simulink model "MoveMoveNewModel"  (R2018a)
settings: Solver=VariableStepAuto  StartTime=0.0  StopTime=10  RelTol=1e-3
PostLoadFcn:
  | helperSetUp
values from neighbouring files (symbols this model uses):
  bf = 12    [data_vehicle.m]    (also in matlab.mat; myVehicle.m)
  br = 14    [data_vehicle.m]    (also in matlab.mat; myVehicle.m)
  Cd = .3    (= 0.3)    [data_vehicle.m]    (also in matlab.mat; myVehicle.m = this.CD)
  Cf = 1.3    [data_vehicle.m]    (also in forwardPropagate.m = 19000; matlab.mat; myVehicle.m; testMotionPlanner.mat = 19000)
  Cr = 1.3    [data_vehicle.m]    (also in forwardPropagate.m = 33000; matlab.mat; myVehicle.m; testMotionPlanner.mat = 33000)
  df = 0.95    [data_vehicle.m]    (also in matlab.mat; myVehicle.m)
  dr = 1    [data_vehicle.m]    (also in matlab.mat; myVehicle.m)
  Ef = -0.1    [data_vehicle.m]    (also in matlab.mat; myVehicle.m)
  Er = -0.1    [data_vehicle.m]    (also in matlab.mat; myVehicle.m)
  fv = .02    (= 0.02)    [data_vehicle.m]    (also in matlab.mat; myVehicle.m)
  Fzf = m*g*lr/l    (= 9879.29185185)    [data_vehicle.m]    (also in matlab.mat; myVehicle.m = m*g*lr/l)
  Fzr = m*g*lf/l    (= 5811.34814815)    [data_vehicle.m]    (also in matlab.mat; myVehicle.m = m*g*lf/l)
  g = 9.80665    [data_vehicle.m]    (also in matlab.mat)
  gB = 2/3    (= 0.666666666667)    [data_vehicle.m]    (also in matlab.mat; myVehicle.m)
  gT = 0    [data_vehicle.m]    (also in matlab.mat; myVehicle.m)
  Jz = 2200    [data_vehicle.m]    (also in matlab.mat; myVehicle.m)
  lf = 1    [data_vehicle.m]    (also in forwardPropagate.m = 1.2; matlab.mat; myVehicle.m; testMotionPlanner.mat = 1.2)
  lr = l-lf    (= 1.7)    [data_vehicle.m]    (also in forwardPropagate.m = 1.6; matlab.mat; myVehicle.m; testMotionPlanner.mat = 1.6)
  m = 1600    [data_vehicle.m]    (also in forwardPropagate.m = 1575; matlab.mat; myVehicle.m; testMotionPlanner.mat = 1575)
  mu = 1    [data_vehicle.m]    (also in matlab.mat; myVehicle.m)
  psi0 = 0    [data_vehicle.m]    (also in matlab.mat)
  psip0 = 0    [data_vehicle.m]    (also in matlab.mat)
  rho = 1.2    [data_vehicle.m]    (also in matlab.mat; myVehicle.m = 1.29)
  S = 2    [data_vehicle.m]    (also in matlab.mat; myVehicle.m)
  vy0 = 0    [data_vehicle.m]    (also in matlab.mat)
  XG0 = 0    [data_vehicle.m]    (also in matlab.mat)
  YG0 = 0    [data_vehicle.m]    (also in matlab.mat)
undefined symbols (not defined in the file or in its folder): deltah, dt_save, fxh
settings Model: Creator=jdrjk  LastModifiedBy=jdrjk

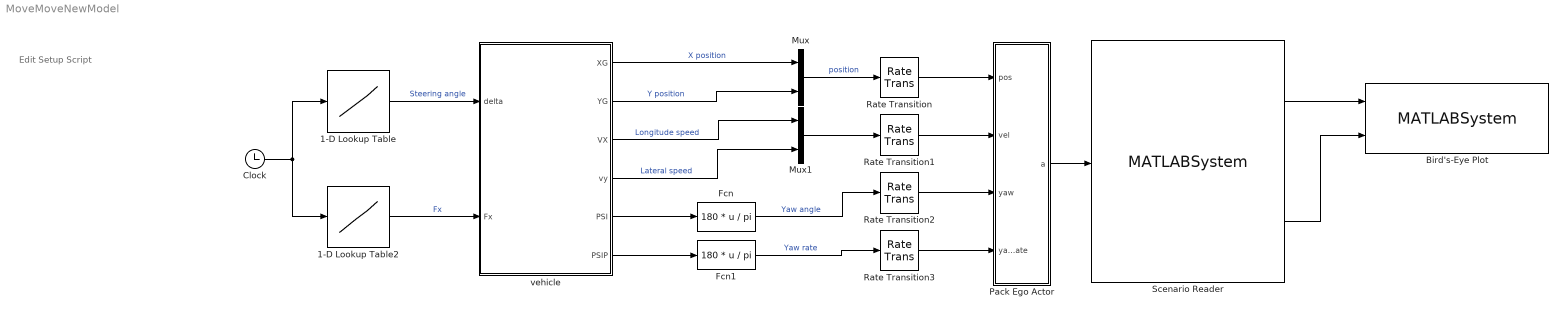
== system MoveMoveNewModel ==
  note: Edit Setup Script
  1-D Lookup Table : Lookup_n-D  NumberOfTableDimensions=1  BreakpointsForDimension1=deltah(:,1)  Table=deltah(:,2)  RndMeth=Simplest  InputSameDT=on
  1-D Lookup Table2 : Lookup_n-D  NumberOfTableDimensions=1  BreakpointsForDimension1=fxh(:,1)  Table=fxh(:,2)  RndMeth=Simplest  InputSameDT=on
  Bird's-Eye Plot : MATLABSystem  System=helperBirdsEyePlot  ScenarioFileName=lkaScenarioSimulink  XLim=[-20, 50 ]  YLim=[ -30, 30 ]  HasActors=on  HasVision=off  HasRadar=off  HasTracks=off  TrackPositionSelector=[ 1, 0, 0, 0, 0, 0; 0, 0, 1, 0, 0, 0 ]  TrackVelocitySelector=[ 0, 1, 0, 0, 0, 0; 0, 0, 0, 1, 0, 0 ]  HasMIO=off  HasRoads=off  HasLaneBoundaries=off  HasLaneMarkings=on
      settings: ModelCloseFcn=helperCloseAll(gcb)
      mask Type: helperBirdsEyePlot
      mask Display:
      | disp(['Bird''s-Eye' char(10) 'Plot']);
      | port_label('input',1,'Actors');
      | port_label('input',2,'Lane Markings');
  Clock : Clock
  Fcn : Fcn  Expr=180 * u / pi
  Fcn1 : Fcn  Expr=180 * u / pi
  Mux : Mux  Inputs=2
  Mux1 : Mux  Inputs=2
  Pack Ego Actor : MATLAB Function  TreatAsAtomicUnit=on
  Rate Transition{,1..3} (4 alike) : RateTransition  OutPortSampleTime=Ts
  Scenario Reader : MATLABSystem  System=helperScenarioReader  ScenarioFileName=lkaScenarioSimulink  EgoActorSource=Input port  EgoActorID=1  RoadBoundaries=off  LaneBoundaries=off  AllBoundaries=off  LaneBoundaryDistance=0:0.5:60  LaneBoundaryLocation=inner  CurrentLane=off  NumLanes=off  LaneMarkings=on  BusNameSource=Auto  BusName2Source=Auto  BusName3Source=Auto  SimulateUsing=Interpreted execution
      mask Type: helperScenarioReader
      mask Display:
      | disp(['Scenario' char(10) 'Reader']);
      | port_label('input',1,'Ego Actor');
      | port_label('output',1,'Actors');
      | port_label('output',2,'Lane Markings');
  vehicle : Subsystem
  wires:
  Rate Transition2/1 -> Pack Ego Actor/3(yaw)
  Mux1/1 -> Rate Transition1/1
  Rate Transition/1 -> Pack Ego Actor/1(pos)
  Scenario Reader/1 -> Bird's-Eye Plot/1
  Fcn1/1 -> Rate Transition3/1  "Yaw rate"
  Mux/1 -> Rate Transition/1  "position"
  Pack Ego Actor/1(a) -> Scenario Reader/1
  Rate Transition3/1 -> Pack Ego Actor/4(yawRate)
  Rate Transition1/1 -> Pack Ego Actor/2(vel)
  Fcn/1 -> Rate Transition2/1  "Yaw angle"
  Scenario Reader/2 -> Bird's-Eye Plot/2
  vehicle/6("PSIP ") -> Fcn1/1
  1-D Lookup Table/1 -> vehicle/1(delta)  "Steering angle"
  Clock/1 -> 1-D Lookup Table/1, 1-D Lookup Table2/1
  vehicle/5(PSI) -> Fcn/1
  vehicle/2(YG) -> Mux/2  "Y position"
  vehicle/1(XG) -> Mux/1  "X position"
  vehicle/3(VX) -> Mux1/1  "Longitude speed"
  vehicle/4(vy) -> Mux1/2  "Lateral speed"
  1-D Lookup Table2/1 -> vehicle/2("Fx ")  "Fx"

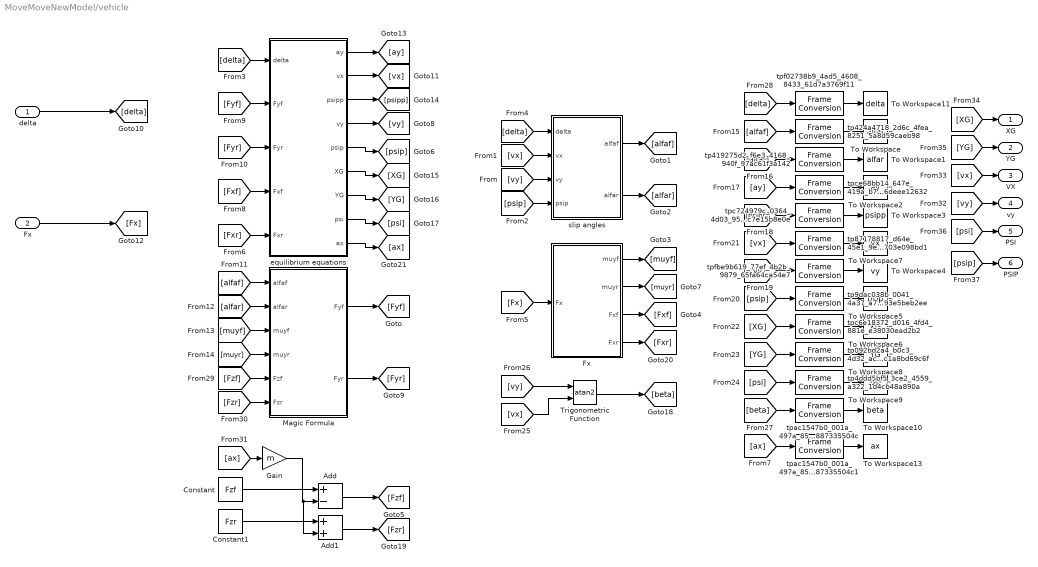
== system MoveMoveNewModel/vehicle ==
  delta : Inport
  "Fx " : Inport  Port=2
  Add : Sum  Inputs=+-
  Add1 : Sum
  Constant : Constant  Value=Fzf
  Constant1 : Constant  Value=Fzr
  Fx : Subsystem
  Gain : Gain  Gain=m
  Magic Formula : Subsystem
  To Workspace : ToWorkspace  VariableName=alfaf  SampleTime=dt_save
  To Workspace1 : ToWorkspace  VariableName=alfar  SampleTime=dt_save
  To Workspace10 : ToWorkspace  VariableName=beta  SampleTime=dt_save
  To Workspace11 : ToWorkspace  VariableName=delta  SampleTime=dt_save
  To Workspace13 : ToWorkspace  VariableName=ax  SampleTime=dt_save
  To Workspace2 : ToWorkspace  VariableName=ay  SampleTime=dt_save
  To Workspace3 : ToWorkspace  VariableName=psipp  SampleTime=dt_save
  To Workspace4 : ToWorkspace  VariableName=vy  SampleTime=dt_save
  To Workspace5 : ToWorkspace  VariableName=psip  SampleTime=dt_save
  To Workspace6 : ToWorkspace  VariableName=XG  SampleTime=dt_save
  To Workspace7 : ToWorkspace  VariableName=vx  SampleTime=dt_save
  To Workspace8 : ToWorkspace  VariableName=YG  SampleTime=dt_save
  To Workspace9 : ToWorkspace  VariableName=psi  SampleTime=dt_save
  Trigonometric Function : Trigonometry  Operator=atan2
  equilibrium equations : Subsystem
  slip angles : Subsystem
  tp092bd2a4_b0c3_4d32_ac59_7c1a8bd69c6f : FrameConversion  OutFrame=Sample-based
  tp419275d2_f6e3_4168_940f_97ac61f3a142 : FrameConversion  OutFrame=Sample-based
  tp424a4718_2d6c_4fea_8251_5a8d59caeb98 : FrameConversion  OutFrame=Sample-based
  tp4ddd5bf5_3ce2_4559_a322_1d4cb48a890a : FrameConversion  OutFrame=Sample-based
  tp87178817_d64e_45e1_9e30_db703e098bd1 : FrameConversion  OutFrame=Sample-based
  tp9dac038b_0041_4a37_a752_0593e5beb2ee : FrameConversion  OutFrame=Sample-based
  tpac1547b0_001a_497a_857c_68887335504c : FrameConversion  OutFrame=Sample-based
  tpac1547b0_001a_497a_857c_68887335504c1 : FrameConversion  OutFrame=Sample-based
  tpc6e18372_d016_4fd4_881e_e38030ead2b2 : FrameConversion  OutFrame=Sample-based
  tpc724979c_0364_4d03_952a_37c7e15b8e0e : FrameConversion  OutFrame=Sample-based
  tpce68bb14_647e_419a_b744_5f6deee12632 : FrameConversion  OutFrame=Sample-based
  tpf02738b9_4ad5_4608_8433_61d7a3769f11 : FrameConversion  OutFrame=Sample-based
  tpfbe9b619_77ef_4b2b_9879_65fa64ca54e7 : FrameConversion  OutFrame=Sample-based
  XG : Outport
  YG : Outport  Port=2
  VX : Outport  Port=3
  vy : Outport  Port=4
  PSI : Outport  Port=5
  "PSIP " : Outport  Port=6
  wires:
  [vx] -> VX/1
  [psi] -> PSI/1
  [XG] -> XG/1
  [YG] -> YG/1
  [vy] -> vy/1
  Magic Formula/2(Fyr) -> [Fyr]
  slip angles/1(alfaf) -> [alfaf]
  equilibrium equations/5(psip) -> [psip]
  [delta] -> equilibrium equations/1(delta)
  [vx] -> slip angles/2(vx)
  Fx/4(Fxr) -> [Fxr]
  [Fxf] -> equilibrium equations/4(Fxf)
  [alfar] -> Magic Formula/2(alfar)
  [muyf] -> Magic Formula/3(muyf)
  [vy] -> slip angles/3(vy)
  [muyr] -> Magic Formula/4(muyr)
  slip angles/2(alfar) -> [alfar]
  Magic Formula/1(Fyf) -> [Fyf]
  [Fyf] -> equilibrium equations/2(Fyf)
  equilibrium equations/4(vy) -> [vy]
  [psip] -> slip angles/4(psip)
  [Fyr] -> equilibrium equations/3(Fyr)
  delta/1 -> [delta]
  Fx/1(muyf) -> [muyf]
  [alfaf] -> Magic Formula/1(alfaf)
  [delta] -> slip angles/1(delta)
  Fx/2(muyr) -> [muyr]
  Fx/3(Fxf) -> [Fxf]
  [delta] -> tpf02738b9_4ad5_4608_8433_61d7a3769f11/1
  tpf02738b9_4ad5_4608_8433_61d7a3769f11/1 -> To Workspace11/1
  [ay] -> tpce68bb14_647e_419a_b744_5f6deee12632/1
  equilibrium equations/8(psi) -> [psi]
  [alfar] -> tp419275d2_f6e3_4168_940f_97ac61f3a142/1
  [alfaf] -> tp424a4718_2d6c_4fea_8251_5a8d59caeb98/1
  tpce68bb14_647e_419a_b744_5f6deee12632/1 -> To Workspace2/1
  [psipp] -> tpc724979c_0364_4d03_952a_37c7e15b8e0e/1
  equilibrium equations/3(psipp) -> [psipp]
  [vy] -> Trigonometric Function/1
  [Fzf] -> Magic Formula/5(Fzf)
  Gain/1 -> Add1/2, Add/2
  tp424a4718_2d6c_4fea_8251_5a8d59caeb98/1 -> To Workspace/1
  [beta] -> tpac1547b0_001a_497a_857c_68887335504c/1
  equilibrium equations/7(YG) -> [YG]
  Add1/1 -> [Fzr]
  tpac1547b0_001a_497a_857c_68887335504c/1 -> To Workspace10/1
  equilibrium equations/1(ay) -> [ay]
  Constant/1 -> Add/1
  equilibrium equations/6(XG) -> [XG]
  Constant1/1 -> Add1/1
  [Fzr] -> Magic Formula/6(Fzr)
  Trigonometric Function/1 -> [beta]
  Add/1 -> [Fzf]
  [vx] -> Trigonometric Function/2
  [ax] -> Gain/1
  tp419275d2_f6e3_4168_940f_97ac61f3a142/1 -> To Workspace1/1
  tp092bd2a4_b0c3_4d32_ac59_7c1a8bd69c6f/1 -> To Workspace8/1
  tp4ddd5bf5_3ce2_4559_a322_1d4cb48a890a/1 -> To Workspace9/1
  tpc724979c_0364_4d03_952a_37c7e15b8e0e/1 -> To Workspace3/1
  [psip] -> tp9dac038b_0041_4a37_a752_0593e5beb2ee/1
  tp87178817_d64e_45e1_9e30_db703e098bd1/1 -> To Workspace7/1
  tpc6e18372_d016_4fd4_881e_e38030ead2b2/1 -> To Workspace6/1
  [vy] -> tpfbe9b619_77ef_4b2b_9879_65fa64ca54e7/1
  tpfbe9b619_77ef_4b2b_9879_65fa64ca54e7/1 -> To Workspace4/1
  [XG] -> tpc6e18372_d016_4fd4_881e_e38030ead2b2/1
  [YG] -> tp092bd2a4_b0c3_4d32_ac59_7c1a8bd69c6f/1
  [vx] -> tp87178817_d64e_45e1_9e30_db703e098bd1/1
  tp9dac038b_0041_4a37_a752_0593e5beb2ee/1 -> To Workspace5/1
  [psi] -> tp4ddd5bf5_3ce2_4559_a322_1d4cb48a890a/1
  [psip] -> "PSIP "/1
  "Fx "/1 -> [Fx]
  [Fx] -> Fx/1(Fx)
  [Fxr] -> equilibrium equations/5("Fxr ")
  equilibrium equations/9(ax) -> [ax]
  [ax] -> tpac1547b0_001a_497a_857c_68887335504c1/1
  tpac1547b0_001a_497a_857c_68887335504c1/1 -> To Workspace13/1
  equilibrium equations/2("vx ") -> [vx]

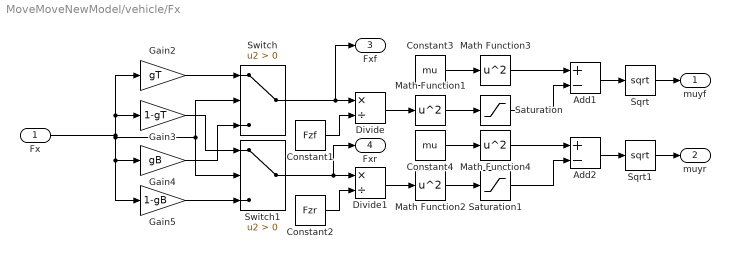
== system MoveMoveNewModel/vehicle/Fx ==
  Fx : Inport
  Add1 : Sum  Inputs=+-
  Add2 : Sum  Inputs=+-
  Constant1 : Constant  Value=Fzf
  Constant2 : Constant  Value=Fzr
  Constant3 : Constant  Value=mu
  Constant4 : Constant  Value=mu
  Divide : Product  Inputs=*/
  Divide1 : Product  Inputs=*/
  Gain2 : Gain  Gain=gT
  Gain3 : Gain  Gain=1-gT
  Gain4 : Gain  Gain=gB
  Gain5 : Gain  Gain=1-gB
  Math Function{1..4} (4 alike) : Math  Operator=square  SaturateOnIntegerOverflow=on
  Saturation : Saturate  UpperLimit=1  LowerLimit=0
  Saturation1 : Saturate  UpperLimit=1  LowerLimit=0
  Sqrt : Sqrt  SaturateOnIntegerOverflow=on
  Sqrt1 : Sqrt  SaturateOnIntegerOverflow=on
  Switch : Switch  Criteria=u2 > Threshold
  Switch1 : Switch  Criteria=u2 > Threshold
  muyf : Outport
  muyr : Outport  Port=2
  Fxf : Outport  Port=3
  Fxr : Outport  Port=4
  wires:
  Gain4/1 -> Switch/3
  Fx/1 -> Gain2/1, Gain3/1, Gain5/1, Gain4/1, Switch1/2, Switch/2
  Gain3/1 -> Switch1/1
  Gain5/1 -> Switch1/3
  Gain2/1 -> Switch/1
  Switch/1 -> Fxf/1, Divide/1
  Switch1/1 -> Fxr/1, Divide1/1
  Constant1/1 -> Divide/2
  Constant2/1 -> Divide1/2
  Constant3/1 -> Math Function3/1
  Divide/1 -> Math Function1/1
  Divide1/1 -> Math Function2/1
  Math Function1/1 -> Saturation/1
  Math Function2/1 -> Saturation1/1
  Constant4/1 -> Math Function4/1
  Saturation1/1 -> Add2/2
  Saturation/1 -> Add1/2
  Add1/1 -> Sqrt/1
  Add2/1 -> Sqrt1/1
  Sqrt1/1 -> muyr/1
  Sqrt/1 -> muyf/1
  Math Function3/1 -> Add1/1
  Math Function4/1 -> Add2/1

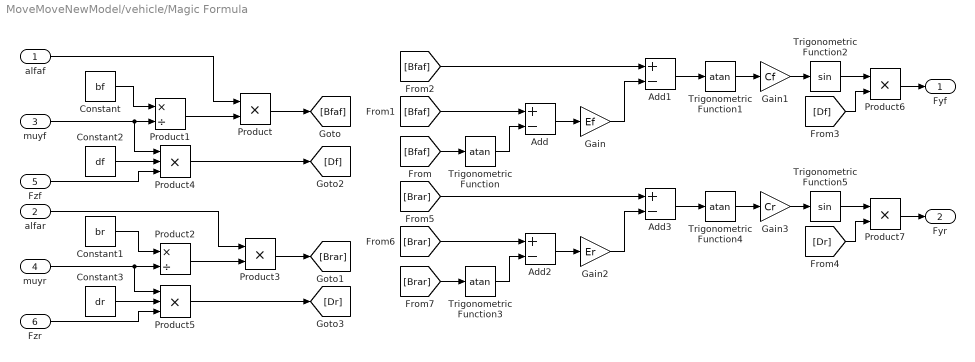
== system MoveMoveNewModel/vehicle/Magic Formula ==
  alfaf : Inport
  alfar : Inport  Port=2
  muyf : Inport  Port=3
  muyr : Inport  Port=4
  Fzf : Inport  Port=5
  Fzr : Inport  Port=6
  Add{,1..3} (4 alike) : Sum  Inputs=+-
  Constant : Constant  Value=bf
  Constant1 : Constant  Value=br
  Constant2 : Constant  Value=df
  Constant3 : Constant  Value=dr
  Gain : Gain  Gain=Ef
  Gain1 : Gain  Gain=Cf
  Gain2 : Gain  Gain=Er
  Gain3 : Gain  Gain=Cr
  Product{,3,6..7} (4 alike) : Product
  Product1 : Product  Inputs=*/
  Product2 : Product  Inputs=*/
  Product4 : Product  Inputs=3
  Product5 : Product  Inputs=3
  Trigonometric Function{,1,3..4} (4 alike) : Trigonometry  Operator=atan
  Trigonometric Function2 : Trigonometry
  Trigonometric Function5 : Trigonometry
  Fyf : Outport
  Fyr : Outport  Port=2
  wires:
  Constant/1 -> Product1/1
  muyf/1 -> Product4/1, Product1/2
  Constant1/1 -> Product2/1
  muyr/1 -> Product5/1, Product2/2
  Product1/1 -> Product/2
  alfaf/1 -> Product/1
  Product2/1 -> Product3/2
  alfar/1 -> Product3/1
  Product/1 -> [Bfaf]
  Product3/1 -> [Brar]
  Constant2/1 -> Product4/2
  Constant3/1 -> Product5/2
  Product4/1 -> [Df]
  Product5/1 -> [Dr]
  [Bfaf] -> Trigonometric Function/1
  Trigonometric Function/1 -> Add/2
  [Bfaf] -> Add/1
  Add/1 -> Gain/1
  Gain/1 -> Add1/2
  [Bfaf] -> Add1/1
  Add1/1 -> Trigonometric Function1/1
  Trigonometric Function1/1 -> Gain1/1
  Gain1/1 -> Trigonometric Function2/1
  Trigonometric Function2/1 -> Product6/1
  [Df] -> Product6/2
  Product6/1 -> Fyf/1
  [Dr] -> Product7/2
  Trigonometric Function5/1 -> Product7/1
  Gain3/1 -> Trigonometric Function5/1
  Trigonometric Function4/1 -> Gain3/1
  Add3/1 -> Trigonometric Function4/1
  [Brar] -> Add3/1
  Gain2/1 -> Add3/2
  Add2/1 -> Gain2/1
  [Brar] -> Add2/1
  Trigonometric Function3/1 -> Add2/2
  [Brar] -> Trigonometric Function3/1
  Product7/1 -> Fyr/1
  Fzf/1 -> Product4/3
  Fzr/1 -> Product5/3

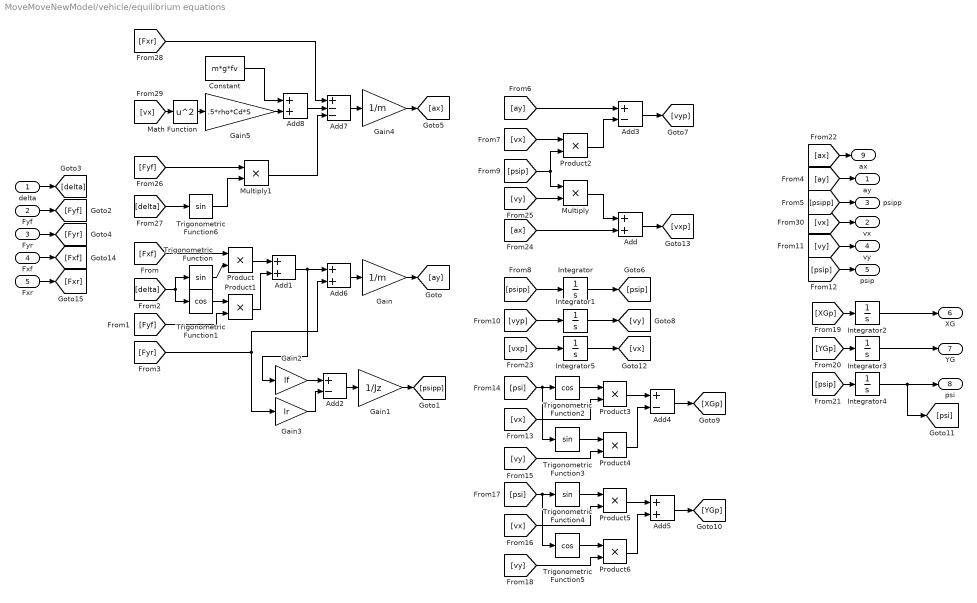
== system MoveMoveNewModel/vehicle/equilibrium equations ==
  delta : Inport
  Fyf : Inport  Port=2
  Fyr : Inport  Port=3
  Fxf : Inport  Port=4
  "Fxr " : Inport  Port=5
  Add{,1,5..6,8} (5 alike) : Sum
  Add2 : Sum  Inputs=+-
  Add3 : Sum  Inputs=+-
  Add4 : Sum  Inputs=+-
  Add7 : Sum  Inputs=+--
  Constant : Constant  Value=m*g*fv
  Gain : Gain  Gain=1/m
  Gain1 : Gain  Gain=1/Jz
  Gain2 : Gain  Gain=lf
  Gain3 : Gain  Gain=lr
  Gain4 : Gain  Gain=1/m
  Gain5 : Gain  Gain=.5*rho*Cd*S
  Integrator : Integrator  InitialCondition=psip0  ContinuousStateAttributes='yaw_rate'
  Integrator1 : Integrator  InitialCondition=vy0  ContinuousStateAttributes='speed_y'
  Integrator2 : Integrator  InitialCondition=XG0  ContinuousStateAttributes='XG'
  Integrator3 : Integrator  InitialCondition=YG0  ContinuousStateAttributes='YG'
  Integrator4 : Integrator  InitialCondition=psi0  ContinuousStateAttributes='yaw'
  Integrator5 : Integrator  InitialCondition=vy0  ContinuousStateAttributes='speed_y'
  Math Function : Math  Operator=square  SaturateOnIntegerOverflow=on
  Multiply : Product
  Multiply1 : Product
  Product{,1..6} (7 alike) : Product
  Trigonometric Function{,3..4,6} (4 alike) : Trigonometry
  Trigonometric Function1 : Trigonometry  Operator=cos
  Trigonometric Function2 : Trigonometry  Operator=cos
  Trigonometric Function5 : Trigonometry  Operator=cos
  ay : Outport
  "vx " : Outport  Port=2
  psipp : Outport  Port=3
  vy : Outport  Port=4
  psip : Outport  Port=5
  XG : Outport  Port=6
  YG : Outport  Port=7
  psi : Outport  Port=8
  ax : Outport  Port=9
  wires:
  Product1/1 -> Add1/2
  Trigonometric Function/1 -> Product/2
  Add6/1 -> Gain/1
  Gain1/1 -> [psipp]
  [Fyr] -> Add6/2, Gain3/1
  Product/1 -> Add1/1
  Gain/1 -> [ay]
  [delta] -> Trigonometric Function/1, Trigonometric Function1/1
  Trigonometric Function1/1 -> Product1/1
  delta/1 -> [delta]
  [ay] -> ay/1
  [Fxf] -> Product/1
  Add1/1 -> Gain2/1, Add6/1
  Fyf/1 -> [Fyf]
  Add2/1 -> Gain1/1
  [Fyf] -> Product1/2
  Gain3/1 -> Add2/2
  Gain2/1 -> Add2/1
  Fyr/1 -> [Fyr]
  [psipp] -> psipp/1
  [psipp] -> Integrator/1
  Integrator/1 -> [psip]
  [vx] -> Product2/1
  [psip] -> Product2/2, Multiply/1
  [ay] -> Add3/1
  Product2/1 -> Add3/2
  Add3/1 -> [vyp]
  [vyp] -> Integrator1/1
  Integrator1/1 -> [vy]
  [vy] -> vy/1
  [psip] -> psip/1
  [psi] -> Trigonometric Function3/1, Trigonometric Function2/1
  Trigonometric Function2/1 -> Product3/1
  [vx] -> Product3/2
  Product3/1 -> Add4/1
  Trigonometric Function3/1 -> Product4/1
  [vy] -> Product4/2
  Product4/1 -> Add4/2
  Add4/1 -> [XGp]
  Add5/1 -> [YGp]
  Product6/1 -> Add5/2
  [vy] -> Product6/2
  Trigonometric Function5/1 -> Product6/1
  Product5/1 -> Add5/1
  [vx] -> Product5/2
  Trigonometric Function4/1 -> Product5/1
  [psi] -> Trigonometric Function4/1, Trigonometric Function5/1
  [XGp] -> Integrator2/1
  Integrator2/1 -> XG/1
  Integrator3/1 -> YG/1
  [YGp] -> Integrator3/1
  Integrator4/1 -> [psi], psi/1
  [psip] -> Integrator4/1
  Fxf/1 -> [Fxf]
  [ax] -> ax/1
  [vxp] -> Integrator5/1
  Integrator5/1 -> [vx]
  Add/1 -> [vxp]
  [vy] -> Multiply/2
  [ax] -> Add/2
  Multiply/1 -> Add/1
  "Fxr "/1 -> [Fxr]
  [delta] -> Trigonometric Function6/1
  Gain4/1 -> [ax]
  [Fyf] -> Multiply1/1
  Trigonometric Function6/1 -> Multiply1/2
  Add7/1 -> Gain4/1
  Multiply1/1 -> Add7/3
  [Fxr] -> Add7/1
  Math Function/1 -> Gain5/1
  [vx] -> Math Function/1
  Gain5/1 -> Add8/2
  Constant/1 -> Add8/1
  Add8/1 -> Add7/2
  [vx] -> "vx "/1

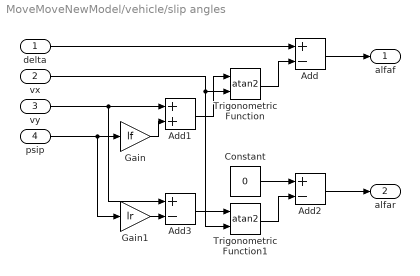
== system MoveMoveNewModel/vehicle/slip angles ==
  delta : Inport
  vx : Inport  Port=2
  vy : Inport  Port=3
  psip : Inport  Port=4
  Add : Sum  Inputs=+-
  Add1 : Sum
  Add2 : Sum  Inputs=+-
  Add3 : Sum  Inputs=+-
  Constant : Constant  Value=0
  Gain : Gain  Gain=lf
  Gain1 : Gain  Gain=lr
  Trigonometric Function : Trigonometry  Operator=atan2
  Trigonometric Function1 : Trigonometry  Operator=atan2
  alfaf : Outport
  alfar : Outport  Port=2
  wires:
  vy/1 -> Add3/1, Add1/1
  Constant/1 -> Add2/1
  Add3/1 -> Trigonometric Function1/1
  Trigonometric Function/1 -> Add/2
  Gain1/1 -> Add3/2
  vx/1 -> Trigonometric Function1/2, Trigonometric Function/2
  psip/1 -> Gain1/1, Gain/1
  Add1/1 -> Trigonometric Function/1
  Gain/1 -> Add1/2
  Trigonometric Function1/1 -> Add2/2
  delta/1 -> Add/1
  Add/1 -> alfaf/1
  Add2/1 -> alfar/1

== matlab function MoveMoveNewModel/Pack Ego Actor ==
  data: pos input; a output Bus: BusActors1Actors size=1; vel input; yaw input; yawRate input
function a = packEgo(pos,vel,yaw,yawRate)
% Pack ego information into a single ego actor bus
%
% Imoprtant note:
% Output is a bus of type BusActorsActors. This is the same bus used by the
% helperScenarioReader to output an individual actor. If you change the
% output bus name of helperScenarioReader, change the output bus name here
% as well by clicking on 'Edit Data' in the menu above.

a = struct(...
    'ActorID',1,...
    'Position', [pos(1) pos(2) 0], ...
    'Velocity', [vel(1) vel(2) 0], ...
    'Roll', 0, ...
    'Pitch', 0, ...
    'Yaw', yaw, ...
    'AngularVelocity', [0 0 yawRate]);
